simulink model "reaction_wheel_control_ss"  (R2023a)
settings: Solver=VariableStepAuto  StartTime=0.0  StopTime=10.0  RelTol=1e-3
values from neighbouring files (symbols this model uses):
  A = [0   1     0   0 ... (first row only)    [model.m]    (also in model_react_wheel_pend2.m = [0   1   0   0)
  B = [0 ... (first row only)    [model.m]    (also in model_react_wheel_pend2.m)
  C = [1 0 0 0 ... (first row only)    [model.m]    (also in model_react_wheel_pend2.m)
  D = [0;0;0;0]    [model.m]    (also in model_react_wheel_pend2.m)
  K = lqrd(A, B, Q, Re, Ts)    [model_react_wheel_pend2.m]
  x0 = [0.2; 0; 0; 0]    [model.m]    (also in model_react_wheel_pend2.m = [3; 0; 0; 0])
settings Model: Creator=skakd  LastModifiedBy=sasha
settings ModelReferenceCC: EnableRefExpFcnMdlSchedulingChecks=on

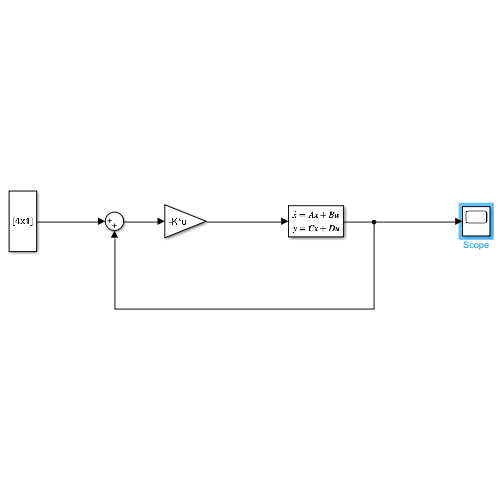
[thumbnail: Simulink's stored preview of the top-level diagram]
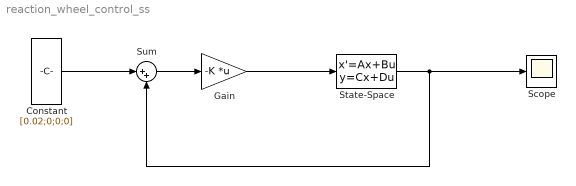
== system reaction_wheel_control_ss ==
  Constant : Constant  Value=[0.02;0;0;0]  VectorParams1D=off
  Gain : Gain  Gain=-K  Multiplication=Matrix(K*u)
  Scope : Scope
  State-Space : StateSpace  A=A  B=B  C=C  D=D  InitialCondition=x0
  Sum : Sum  Inputs=|++
  wires:
  Sum/1 -> Gain/1
  Constant/1 -> Sum/1
  State-Space/1 -> Scope/1, Sum/2
  Gain/1 -> State-Space/1
